simulink model "MPModel_gl"  (R2013a)
settings: Solver=FixedStepDiscrete  StartTime=0.0  StopTime=5  FixedStep=0.01  RelTol=1e-3
settings Model: Creator=Admin  LastModifiedBy=nadarge
settings DataIOCC: LimitDataPoints=off

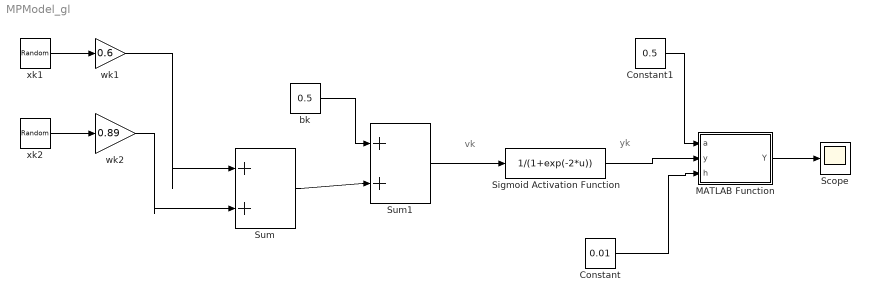
== system MPModel_gl ==
  note: yk
  note: vk
  Constant : Constant  Value=0.01
  Constant1 : Constant  Value=0.5
  MATLAB Function : MATLAB Function  TreatAsAtomicUnit=on
  Scope : Scope
  Sigmoid Activation Function : Fcn  Expr=1/(1+exp(-2*u))
  Sum : Sum  Inputs=|++
  Sum1 : Sum  Inputs=|++
  bk : Constant  Value=0.5
  wk1 : Gain  Gain=0.6
  wk2 : Gain  Gain=0.89
  xk1 : RandomNumber  SampleTime=0
  xk2 : RandomNumber  SampleTime=0
  wires:
  xk1/1 -> wk1/1
  xk2/1 -> wk2/1
  wk1/1 -> Sum/1
  wk2/1 -> Sum/2
  bk/1 -> Sum1/1
  Sum/1 -> Sum1/2
  Sum1/1 -> Sigmoid Activation Function/1
  Sigmoid Activation Function/1 -> MATLAB Function/2(y)
  Constant1/1 -> MATLAB Function/1(a)
  Constant/1 -> MATLAB Function/3(h)
  MATLAB Function/1(Y) -> Scope/1

== matlab function MPModel_gl/MATLAB Function ==
  data: a input; y input; h input; Y output
function Y = fgl_deriv( a, y, h )
%#codegen

 n  = numel(y);
    J  = 0:(n-1);
    G1 = gamma( J+1 );
    G2 = gamma( a+1-J );
    s  = (-1) .^ J;

    M  = tril( ones(n) );
    R  = toeplitz( y(:)' );
    T  = meshgrid( (gamma(a+1)/(h^a)) * s ./ (G1.*G2) );
    Y  = reshape(sum( R .* M .* T, 2 ), size(y));
    
    
end
